simulink model "Offline_MiL_Sim_Public"  (R2024a)
settings: Solver=ode1  StartTime=0.0  StopTime=inf  FixedStep=step_size  RelTol=1e-3  EnableMultiTasking=on
PostLoadFcn:
  | if any(exist('dsrtsu_mdlpostloadfcn', 'file') ~= 0), dsrtsu_mdlpostloadfcn('Execute', bdroot); end
InitFcn:
  | , if any(exist('rtifpga_mdlclblib', 'file') ~= 0), rtifpga_mdlclblib('Init', bdroot); end,
  | , if any(exist('dsmpb_private', 'file') ~= 0), dsmpb_private('dsmpb_mdlclblib', 'Init', bdroot); end,
undefined symbols (not defined in the file or in its folder): Af, break_criteria, C_r, C_w, Cd, CurrentLosses, dens, DiscIntNeverNeededParam, FDR, fr, Friction, gain_Twr, grade_track, grav, IronLosses, Kp_c, lbh_ac, lbx_ac, lbx_ac_e, lbx_mhe, M_EM_acc_0, M_EM_acc_max, M_EM_brk_min, M_gen_max, M_mot_max, mpc_init_EM_acc, mpc_init_EM_brk, mpc_init_fric_brk, mps_kmh, Mv, n_0, n_em_max, n_gen_max, n_mot_max, n_vec, nout, numHiddenUnits, options, options_mhe, optparam, P, parameter_0, Q, R, r_dyn, R_w_c, R_w_e, R_w_r, rps_rpm, s_track, SE_selector_sim, start_distance_check, step_size, T_c, T_cool, T_e, T_init, T_max, t_mpc_on, T_r_0 ... (+21)
libraries: simulink x3, matrix_library x2, deeplib x1
(part 2 of 2)

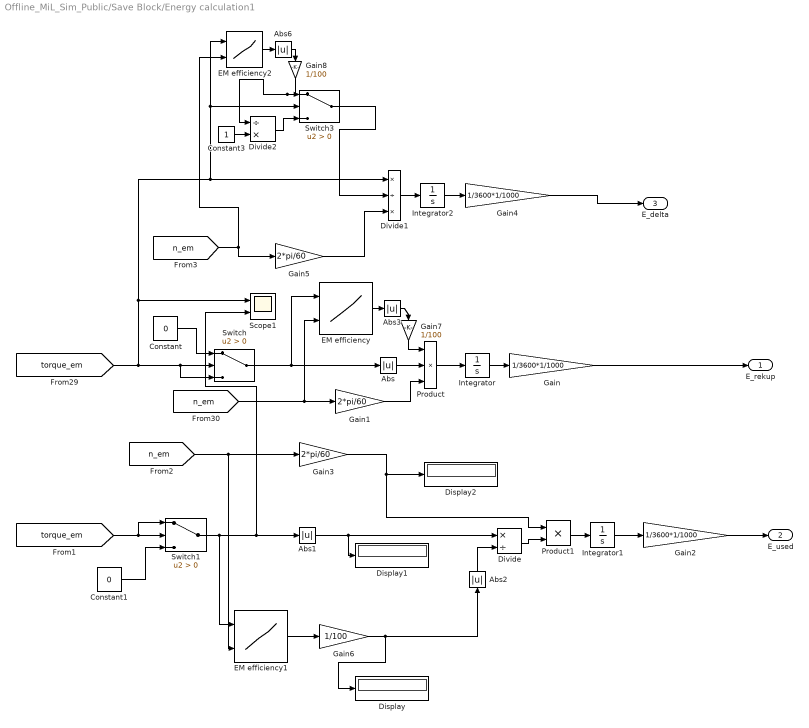
== system Offline_MiL_Sim_Public/Save Block/Energy calculation1 ==
  Abs{,1..3,6} (5 alike) : Abs  SaturateOnIntegerOverflow=off
  Constant : Constant  Value=0
  Constant1 : Constant  Value=0
  Constant3 : Constant
  Display : Display
  Display1 : Display
  Display2 : Display
  Divide : Product  Inputs=*/
  Divide1 : Product  Inputs=*/*
  Divide2 : Product  Inputs=/*
  EM efficiency : Lookup_n-D  BreakpointsForDimension1=data_efficiency(2:end,1)  BreakpointsForDimension2=data_efficiency(1,2:end)  Table=data_efficiency(2:end,2:end)  InternalRulePriority=Speed  RndMeth=Simplest
      settings: InputPortMap=u0,u1
  EM efficiency1 : Lookup_n-D  BreakpointsForDimension1=data_efficiency(2:end,1)  BreakpointsForDimension2=data_efficiency(1,2:end)  Table=data_efficiency(2:end,2:end)  InternalRulePriority=Speed  RndMeth=Simplest
      settings: InputPortMap=u0,u1
  EM efficiency2 : Lookup_n-D  BreakpointsForDimension1=data_efficiency(2:end,1)  BreakpointsForDimension2=data_efficiency(1,2:end)  Table=data_efficiency(2:end,2:end)  InternalRulePriority=Speed  RndMeth=Simplest
      settings: InputPortMap=u0,u1
  Gain : Gain  Gain=1/3600*1/1000
  Gain1 : Gain  Gain=2*pi/60
  Gain2 : Gain  Gain=1/3600*1/1000
  Gain3 : Gain  Gain=2*pi/60
  Gain4 : Gain  Gain=1/3600*1/1000
  Gain5 : Gain  Gain=2*pi/60
  Gain6 : Gain  Gain=1/100
  Gain7 : Gain  Gain=1/100
  Gain8 : Gain  Gain=1/100
  Integrator : Integrator
  Integrator1 : Integrator
  Integrator2 : Integrator
  Product : Product  Inputs=3
  Product1 : Product
  Scope1 : Scope  NumInputPorts=2
  Switch : Switch  Criteria=u2 > Threshold  SaturateOnIntegerOverflow=off  InputSameDT=off
  Switch1 : Switch  Criteria=u2 > Threshold  SaturateOnIntegerOverflow=off  InputSameDT=off
  Switch3 : Switch  Criteria=u2 > Threshold  SaturateOnIntegerOverflow=off  InputSameDT=off
  E_rekup : Outport  VectorParamsAs1DForOutWhenUnconnected=off
  E_used : Outport  Port=2  VectorParamsAs1DForOutWhenUnconnected=off
  E_delta : Outport  Port=3  VectorParamsAs1DForOutWhenUnconnected=off
  wires:
  Product/1 -> Integrator/1
  Switch/1 -> EM efficiency/1, Abs/1
  Gain1/1 -> Product/3
  Abs3/1 -> Gain7/1
  [n_em] -> Gain1/1, EM efficiency/2
  Abs/1 -> Product/2
  Constant/1 -> Switch/1
  Gain/1 -> E_rekup/1
  Integrator/1 -> Gain/1
  Divide/1 -> Product1/2
  Switch1/1 -> Scope1/2, Abs1/1, EM efficiency1/1
  [n_em] -> Gain3/1, EM efficiency1/2
  Abs1/1 -> Display1/1, Divide/1
  [torque_em] -> Switch1/1, Switch1/2
  Constant1/1 -> Switch1/3
  Gain2/1 -> E_used/1
  Integrator1/1 -> Gain2/1
  Product1/1 -> Integrator1/1
  Gain3/1 -> Product1/1, Display2/1
  Abs2/1 -> Divide/2
  EM efficiency/1 -> Abs3/1
  Integrator2/1 -> Gain4/1
  Gain4/1 -> E_delta/1
  Divide1/1 -> Integrator2/1
  [torque_em] -> Divide1/1, Switch3/2, EM efficiency2/1, Scope1/1, Switch/3, Switch/2
  [n_em] -> EM efficiency2/2, Gain5/1
  EM efficiency2/1 -> Abs6/1
  Gain5/1 -> Divide1/3
  Switch3/1 -> Divide1/2
  Abs6/1 -> Gain8/1
  Divide2/1 -> Switch3/3
  Constant3/1 -> Divide2/2
  Gain6/1 -> Display/1, Abs2/1
  EM efficiency1/1 -> Gain6/1
  Gain8/1 -> Divide2/1, Switch3/1
  Gain7/1 -> Product/1

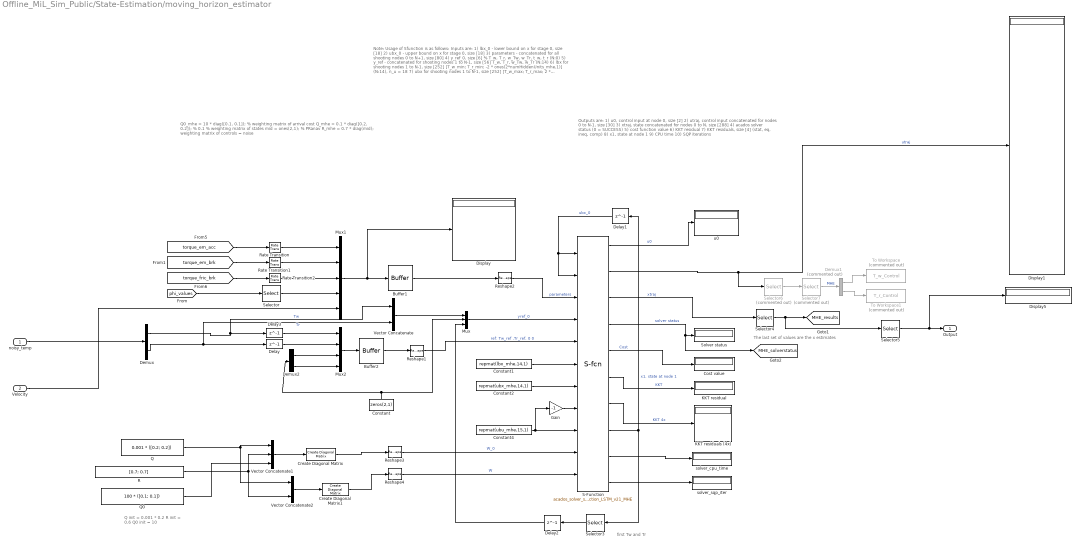
== system Offline_MiL_Sim_Public/State-Estimation/moving_horizon_estimator ==
  note: first Tw and Tr
  note: Q0_mhe = 10 * diag([0.1, 0.1]); % weighting matrix of arrival cost
      | Q_mhe = 0.1 * diag([0.2, 0.2]); % 0.1 % weighting matrix of states
      | mid = ones(2,1); % PRanav
      | R_mhe = 0.7 * diag(mid); weighting matrix of controls = noise
  note: Q init = 0.001 * 0.2
      | R init = 0.6
      | Q0 init = 10
  note: The last set of values are the x estimates
  note: Outputs are:
      | 1) u0, control input at node 0, size [2]
      | 2) utraj, control input concatenated for nodes 0 to N-1, size [30]
      | 3) xtraj, state concatenated for nodes 0 to N, size [288]
      | 4) acados solver status (0 = SUCCESS)
      | 5) cost function value
      | 6) KKT residual
      | 7) KKT residuals, size [4] (stat, eq, ineq, comp)
      | 8) x1, state at node 1
      | 9) CPU time
      | 10) SQP iterations
  note: Note: Usage of Sfunction is as follows:
      | Inputs are:
      | 1) lbx_0 - lower bound on x for stage 0, size [18]
      | 2) ubx_0 - upper bound on x for stage 0, size [18]
      | 3) parameters - concatenated for all shooting nodes 0 to N+1, size [80]
      | 4) y_ref_0, size [6]
      | % T_w, T_r, w_Tw, w_Tr, t_w, t_r (N:0)
      | 5) y_ref - concatenated for shooting nodes 1 to N-1, size [56]
      | T_w, T_r, w_Tw, w_Tr (N:14)
      | 6) lbx for shooting nodes 1 to N-1, size [252]
      | [T_w_min; T_r_min; -2 * ones(2*numHiddenUnits_mhe,1)] (N:14), n_u = 18
      | 7) ubx for shooting nodes 1 to N-1, size [252]
      | [T_w_max; T_r_max; 2 * ones(2*numHiddenUnits_mhe,1)] (N:14), n_u = 18
      | 8) lbu for shooting nodes 0 to N-1, size [30]
      | [0; 0] (N:15)
      | 9) ubu for shooting nodes 0 to N-1, size [30]
      | [100; 100] (N:15)
      | 10) cost_W_0 in column-major format, size [36]
      | blkdiag(Q_mhe, R_mhe, Q0_mhe)
      | 11) cost_W in column-major format, that is set for all intermediate shooting nodes: 1 to N-1, size [16]
      | blkdiag(Q_mhe, R_mhe)
  noisy_temp : Inport
  Velocity : Inport  Port=2
  Buffer1 : Buffer  N=(options_mhe.P+1)*options_mhe.n_parameter  V=((options_mhe.P+1)*options_mhe.n_parameter)-options_mhe.n_parameter  OutputFrames=off
  Buffer2 : Buffer  N=(options_mhe.P-1)*nout  V=(options_mhe.P-2)*nout  ic=repmat([60;60;0;0],13,1)  OutputFrames=off
  Constant : Constant  Value=zeros(2,1)
  Constant1 : Constant  Value=repmat(lbx_mhe,14,1)  SampleTime=options.Ts
  Constant2 : Constant  Value=repmat(ubx_mhe,14,1)  SampleTime=options.Ts
  Constant4 : Constant  Value=repmat(ubu_mhe,15,1)  SampleTime=options.Ts
  Cost value : Display
  Create Diagonal Matrix : matrix_library/Create Diagonal Matrix
      settings: LibrarySourceBlock=|
      | simulink/Matrix
      | Operations/Create Diagonal
      | Matrix
  Create Diagonal Matrix1 : matrix_library/Create Diagonal Matrix
      settings: LibrarySourceBlock=|
      | simulink/Matrix
      | Operations/Create Diagonal
      | Matrix
  Delay : Delay  DelayLength=1  InitialCondition=60
  Delay1 : Delay  DelayLength=1  InitialCondition=options_mhe.x0
  Delay2 : Delay  DelayLength=1  InitialCondition=[60;60]
  Delay3 : Delay  DelayLength=1  InitialCondition=60
  Demux : Demux  Outputs=2
  Demux1 : Demux  Commented=on  Outputs=2
  Demux2 : Demux  Outputs=2
  Display : Display
  Display1 : Display
  Display5 : Display
  Gain : Gain  Gain=-1
  KKT residual : Display
  KKT residuals (4x) : Display
  Mux : Mux  Inputs=3
  Mux1 : Mux  Inputs=5
  Mux2 : Mux
  Q : Constant  Value=0.001 * ([0.2; 0.2])  VectorParams1D=off
  Q0 : Constant  Value=100 * ([0.1; 0.1])
  R : Constant  Value=[0.7; 0.7]
  Rate Transition : RateTransition  OutPortSampleTime=options_mhe.Ts
  Rate Transition1 : RateTransition  OutPortSampleTime=options_mhe.Ts
  Rate Transition2 : RateTransition  OutPortSampleTime=options_mhe.Ts
  Reshape{1..4} (4 alike) : Reshape
  S-Function : S-Function  FunctionName=acados_solver_sfunction_LSTM_v21_MHE  SFunctionDeploymentMode=off  EnableBusSupport=off
  Selector : Selector  InputPortWidth=41  IndexOptions=Index vector (dialog)  Indices=1  OutputSizes=1
  Selector3 : Selector  InputPortWidth=2+(numHiddenUnits*2)  IndexOptions=Index vector (dialog)  Indices=[1 2]  OutputSizes=1
  Selector4 : Selector  InputPortWidth=288  IndexOptions=Index vector (dialog)  Indices=[(18*15)+1:18*16]  OutputSizes=1
  Selector5 : Selector  InputPortWidth=18  IndexOptions=Index vector (dialog)  Indices=[1 2]  OutputSizes=1
  Selector6 : Selector  Commented=on  InputPortWidth=18*15  IndexOptions=Index vector (dialog)  Indices=[(18*14)+1:18*15]  OutputSizes=1
  Selector7 : Selector  Commented=on  InputPortWidth=18  IndexOptions=Index vector (dialog)  Indices=[1:2]  OutputSizes=1
  Solver status : Display
  To Workspace : ToWorkspace  Commented=on  VariableName=T_w_Control  SampleTime=-1
      settings: Save2DSignal=2-D array (concatenate along first dimension)
  To Workspace1 : ToWorkspace  Commented=on  VariableName=T_r_Control  SampleTime=-1
      settings: Save2DSignal=2-D array (concatenate along first dimension)
  Vector Concatenate : Concatenate
  Vector Concatenate1 : Concatenate  NumInputs=3
  Vector Concatenate2 : Concatenate
  solver_cpu_time : Display
  solver_sqp_iter : Display
  u0 : Display
  Output : Outport
  tag scope: MHE_results=global, MHE_solverstatus=global
  wires:
  [torque_fric_brk] -> Rate Transition2/1
  Mux/1 -> S-Function/4  "yref_0"
  [torque_em_brk] -> Rate Transition1/1
  S-Function/2 -> Display1/1, Selector6/1  "utraj"
  R/1 -> Vector Concatenate1/2, Vector Concatenate2/2
  Velocity/1 -> Mux1/5
  Q0/1 -> Vector Concatenate1/3
  Create Diagonal Matrix1/1 -> Reshape4/1
  S-Function/3 -> Selector4/1  "xtraj"
  noisy_temp/1 -> Demux/1
  [phi_values] -> Selector/1
  Rate Transition2/1 -> Mux1/3
  Demux/2 -> Vector Concatenate/2, Delay/1  "Tr"
  Create Diagonal Matrix/1 -> Reshape3/1
  Buffer1/1 -> Reshape2/1
  Q/1 -> Vector Concatenate1/1, Vector Concatenate2/1
  Vector Concatenate1/1 -> Create Diagonal Matrix/1
  Delay1/1 -> S-Function/2, S-Function/1  "ubx_0"
  Vector Concatenate/1 -> Mux/1
  S-Function/1 -> u0/1  "u0"
  Selector4/1 -> Selector5/1, [MHE_results]
  Demux/1 -> Delay3/1, Vector Concatenate/1  "Tw"
  Vector Concatenate2/1 -> Create Diagonal Matrix1/1
  Reshape2/1 -> S-Function/3  "parameters"
  [torque_em_acc] -> Rate Transition/1
  Rate Transition/1 -> Mux1/1
  Rate Transition1/1 -> Mux1/2
  S-Function/4 -> [MHE_solverstatus], Solver status/1  "solver status"
  Mux1/1 -> Display/1, Buffer1/1
  Selector/1 -> Mux1/4
  Selector5/1 -> Display5/1, Output/1
  Selector6/1 -> Selector7/1
  Selector7/1 -> Demux1/1  "MHE"
  Demux1/1 -> To Workspace/1
  Demux1/2 -> To Workspace1/1
  Reshape4/1 -> S-Function/11  "W"
  Reshape3/1 -> S-Function/10  "W_0"
  Constant1/1 -> S-Function/6
  Constant2/1 -> S-Function/7
  Constant4/1 -> S-Function/9, Gain/1
  Reshape1/1 -> S-Function/5  "ref: Tw_ref ,Tr_ref, 0 0"
  Demux2/1 -> Mux2/3
  Demux2/2 -> Mux2/4
  Delay/1 -> Mux2/2
  Delay3/1 -> Mux2/1
  Mux2/1 -> Buffer2/1
  Buffer2/1 -> Reshape1/1
  S-Function/10 -> solver_sqp_iter/1
  S-Function/9 -> solver_cpu_time/1
  S-Function/5 -> Cost value/1  "Cost"
  S-Function/8 -> Delay1/1, Selector3/1  "x1, state at node 1"
  S-Function/6 -> KKT residual/1  "KKT"
  S-Function/7 -> KKT residuals (4x)/1  "KKT 4x"
  Delay2/1 -> Mux/3
  Constant/1 -> Demux2/1, Mux/2
  Selector3/1 -> Delay2/1
  Gain/1 -> S-Function/8

== system Offline_MiL_Sim_Public/Vehicle Model/Driver Model ==
  note: source: Jinming Liu, Modeling, Configuration and control optimization of power split hybrid vehiclesm, Dissertation, 2007
  v_veh (km/h) : Inport
  v_des (km/h) : Inport  Port=2
  "-1 to 1 " : Saturate  UpperLimit=1  LowerLimit=-1
  1/Ti_c : Gain  Gain=1/Ti_c  SaturateOnIntegerOverflow=on  OutDataTypeStr=Inherit: Same as input  ParamDataTypeStr=Inherit: Same as input
  1/Tt_c : Gain  Gain=1/Tt_c  SaturateOnIntegerOverflow=on  OutDataTypeStr=Inherit: Same as input  ParamDataTypeStr=Inherit: Same as input
  Integrator1 : Integrator
  Kp_c : Gain  Gain=Kp_c  SaturateOnIntegerOverflow=on  OutDataTypeStr=Inherit: Same as input  ParamDataTypeStr=Inherit: Same as input
  Normalize : Gain  Gain=1/v_max_c  SaturateOnIntegerOverflow=on  OutDataTypeStr=Inherit: Same as input  ParamDataTypeStr=Inherit: Same as input
  Normalize1 : Gain  Gain=1/v_max_c  SaturateOnIntegerOverflow=on  OutDataTypeStr=Inherit: Same as input  ParamDataTypeStr=Inherit: Same as input
  Sum1 : Sum  InputSameDT=on  SaturateOnIntegerOverflow=on  OutDataTypeStr=Inherit: Same as first input
  Sum5 : Sum  Inputs=-+  InputSameDT=on  SaturateOnIntegerOverflow=on  OutDataTypeStr=Inherit: Same as first input
  Sum7 : Sum  Inputs=+-  InputSameDT=on  SaturateOnIntegerOverflow=on  OutDataTypeStr=Inherit: Same as first input
  Sum8 : Sum  InputSameDT=on  SaturateOnIntegerOverflow=on  OutDataTypeStr=Inherit: Same as first input
  driver_cmd : Outport  VectorParamsAs1DForOutWhenUnconnected=off
  wires:
  Normalize/1 -> Sum7/1
  v_veh (km/h)/1 -> Normalize1/1  "v_ist"
  v_des (km/h)/1 -> Normalize/1  "vdes"
  Sum5/1 -> 1/Tt_c/1
  "-1 to 1 "/1 -> Sum5/2, driver_cmd/1
  Integrator1/1 -> Sum1/2
  1/Ti_c/1 -> Sum8/1
  Sum8/1 -> Integrator1/1
  1/Tt_c/1 -> Sum8/2
  Kp_c/1 -> 1/Ti_c/1, Sum1/1
  Sum1/1 -> "-1 to 1 "/1, Sum5/1
  Sum7/1 -> Kp_c/1
  Normalize1/1 -> Sum7/2

== system Offline_MiL_Sim_Public/Vehicle Model/LSTM-Based Thermal Model grad ==
  Rotational_Speed [rpm] : Inport
  Torque_EM [Nm] : Inport  Port=2
  Constant3 : Constant  Value=YMin_mhe
  Constant4 : Constant  Value=T_cool
  Delay : Delay  DelayLength=1  InitialCondition=[T_w_0;T_r_0]
  Demux4 : Demux  Outputs=2
  Demux5 : Demux  Commented=on  Outputs=2
  Discrete-Time Integrator : DiscreteIntegrator  gainval=1  InitialCondition=[T_w_0;T_r_0]  SampleTime=-1  ICPrevOutput=DiscIntNeverNeededParam  ICPrevScaledInput=DiscIntNeverNeededParam
  From1 : From  Commented=on  GotoTag=T_wr  TagVisibility=global
  Gain2 : Gain  Gain=1/n_em_max
  Gain3 : Gain  Gain=1/M_EM_acc_max
  Gain6 : Gain  Gain=YMax_mhe-YMin_mhe
  Gain7 : Gain  Gain=1/(T_max-T_cool)
  Gain8 : Gain  Gain=1/(T_max-T_cool)
  Mux : Mux
  Reshape : Reshape  OutputDimensionality=Customize  OutputDimensions=[4,1]
  Stateful Predict : deeplib/Stateful Predict  Network=Network from MAT-file  NetworkFunction=untitled  NetworkFilePath=e_Sim\LSTM_8HU_10000ep_grad_slx.mat  InputDataFormats={ '', '' }  SampleTime=-1  ForceInterpretedSim=off  EnableDLNetwork=on  LastKnownNetworkFilePath=''  LastKnownNetworkTimeStamp=''
  Sum2 : Sum  Inputs=|++
  Sum3 : Sum  Inputs=-+|
  Sum4 : Sum  Inputs=-+|
  To Workspace17 : ToWorkspace  VariableName=XTest  SaveFormat=Timeseries  SampleTime=-1
  To Workspace18 : ToWorkspace  VariableName=YPred  SaveFormat=Timeseries  SampleTime=-1
  T_w_LSTM [°C] : Outport
  T_r_LSTM [°C] : Outport  Port=2
  wires:
  Mux/1 -> Reshape/1
  Demux5/1 -> ?
  Rotational_Speed [rpm]/1 -> Gain2/1
  Torque_EM [Nm]/1 -> Gain3/1
  Gain7/1 -> Mux/3
  Sum4/1 -> Gain8/1
  Stateful Predict/1 -> Gain6/1
  Constant4/1 -> Sum4/1, Sum3/1
  Gain8/1 -> Mux/4
  Sum3/1 -> Gain7/1
  Gain2/1 -> Mux/1
  Demux5/2 -> ?
  Demux4/2 -> Sum4/2, T_r_LSTM [°C]/1
  Delay/1 -> Demux4/1
  Constant3/1 -> Sum2/2
  Demux4/1 -> Sum3/2, T_w_LSTM [°C]/1
  Sum2/1 -> Discrete-Time Integrator/1, To Workspace18/1
  From1/1 -> Demux5/1
  Discrete-Time Integrator/1 -> Delay/1
  Gain3/1 -> Mux/2
  Gain6/1 -> Sum2/1
  Reshape/1 -> Stateful Predict/1, To Workspace17/1

== system Offline_MiL_Sim_Public/Vehicle Model/Thermal Model DENSO ==
  "SpeedIn " : Inport
  TorqueIn : Inport  Port=2
  Ground : Ground
  Terminator : Terminator
  Terminator1 : Terminator
  T_wr : Outport
  T_wr_muxed : Outport  Port=2
  wires:
  TorqueIn/1 -> Terminator/1  "TorqueIn"
  "SpeedIn "/1 -> Terminator1/1
  Ground/1 -> T_wr_muxed/1, T_wr/1

== system Offline_MiL_Sim_Public/Vehicle Model/Thermisches Modell EM - LPTN ==
  Drehzahl_rpm : Inport
  Torque_Nm : Inport  Port=2
  Abs : Abs  SaturateOnIntegerOverflow=off
  Coolant Temp : Constant  Value=T_c  VectorParams1D=off
  Demux : Demux  Outputs=2
  Demux1 : Demux  Outputs=2
  Demux2 : Demux  Outputs=2
  Display : Display
  Display1 : Display
  Display2 : Display
  Environment Temp : Constant  Value=T_e  VectorParams1D=off
  Gain1 : Gain  Gain=0.8
  Gain2 : Gain  Gain=0.2
  Goto : Goto  Commented=on  GotoTag=R_w_r  TagVisibility=global
  Goto1 : Goto  Commented=on  GotoTag=R_r_e  TagVisibility=global
  K->C : Constant  Value=273.15
  "LPTN Model " : Subsystem
  Mux : Mux  Inputs=2
  Mux1 : Mux
  Parameter Calculation : Subsystem  Commented=on
  Subsystem1 : Subsystem
  Subsystem2 : Subsystem
  Subsystem3 : Subsystem
  Sum : Sum  Inputs=|++
  Sum1 : Sum  Inputs=++|
  Sum5 : Sum  Inputs=|+-
  Temperaturen_C : Outport  VectorParamsAs1DForOutWhenUnconnected=off
  wires:
  Demux/1 -> Subsystem3/1(torque)  "torque"
  Demux/2 -> Subsystem3/2(speed)  "speed"
  Demux2/1 -> Subsystem2/1(torque)  "torque"
  Demux2/2 -> Subsystem2/2(speed)  "speed"
  Demux1/1 -> Subsystem1/1(torque)  "torque"
  Demux1/2 -> Subsystem1/2(speed)  "speed"
  Subsystem3/1(iron loss) -> Sum/1
  Sum1/1 -> Display1/1, Mux1/2  "P_R"
  Subsystem2/1(friction loss) -> Sum1/2
  Gain2/1 -> Sum1/1
  Gain1/1 -> Sum/2
  Sum/1 -> Display/1, Mux1/1  "P_W"
  Coolant Temp/1 -> Mux1/3
  Environment Temp/1 -> Mux1/4
  Mux1/1 -> "LPTN Model "/1(1:Pw 2: Pr 3:Tc  4:Te)
  "LPTN Model "/1("1:Tw, 2:Tr") -> Sum5/1  "[K]"
  Subsystem1/1(iron loss) -> Gain1/1, Gain2/1
  Drehzahl_rpm/1 -> Mux/2
  Mux/1 -> Demux2/1, Demux1/1, Demux/1
  K->C/1 -> Sum5/2
  Sum5/1 -> Display2/1, Temperaturen_C/1  "[gradC]"
  Parameter Calculation/1(R_w_r) -> Goto/1
  Parameter Calculation/2(R_r_e) -> Goto1/1
  Torque_Nm/1 -> Abs/1
  Abs/1 -> Mux/1

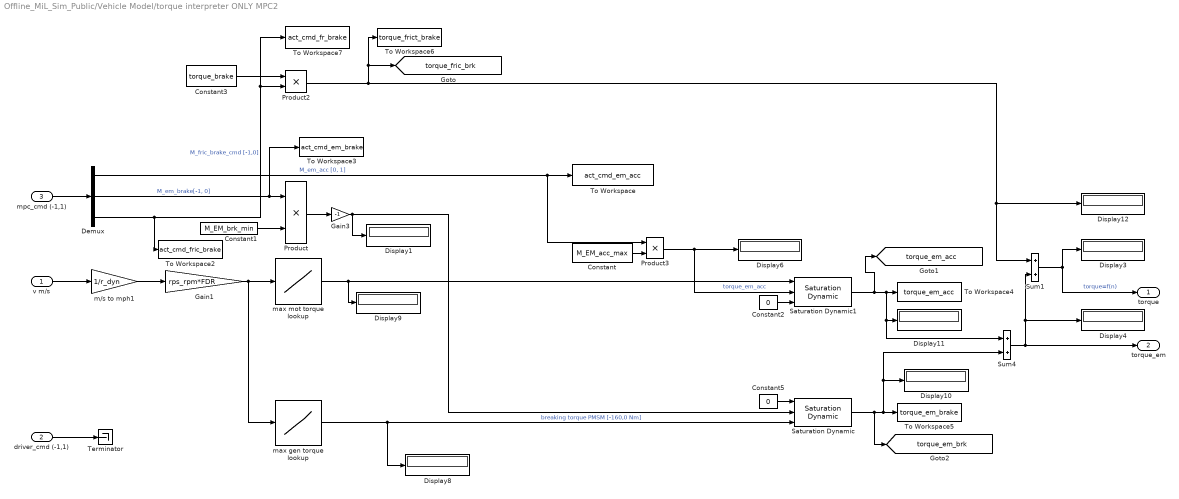
== system Offline_MiL_Sim_Public/Vehicle Model/torque interpreter ONLY MPC2 ==
  v m/s : Inport
  driver_cmd (-1,1) : Inport  Port=2
  mpc_cmd (-1,1) : Inport  Port=3
  Constant : Constant  Value=M_EM_acc_max
  Constant1 : Constant  Value=M_EM_brk_min
  Constant2 : Constant  Value=0
  Constant3 : Constant  Value=torque_brake
  Constant5 : Constant  Value=0
  Demux : Demux  Outputs=3
  Display{1,3..4,6,8..12} (9 alike) : Display
  Gain1 : Gain  Gain=rps_rpm*FDR
  Gain3 : Gain  Gain=-1
  Product : Product
  Product2 : Product
  Product3 : Product
  Saturation Dynamic : simulink/Discontinuities/Saturation Dynamic  OutMin=[]  OutMax=[]  OutDataTypeStr=Inherit: Same as second input  OutDataType=fixdt(1, 16)  OutScaling=2^-10  DoSatur=off
  Saturation Dynamic1 : simulink/Discontinuities/Saturation Dynamic  OutMin=[]  OutMax=[]  OutDataTypeStr=Inherit: Same as second input  OutDataType=fixdt(1, 16)  OutScaling=2^-10  DoSatur=off
  Sum1 : Sum
  Sum4 : Sum
  Terminator : Terminator
  To Workspace : ToWorkspace  VariableName=act_cmd_em_acc  SampleTime=-1
      settings: Save2DSignal=2-D array (concatenate along first dimension)
  To Workspace2 : ToWorkspace  VariableName=act_cmd_fric_brake  SampleTime=-1
      settings: Save2DSignal=2-D array (concatenate along first dimension)
  To Workspace3 : ToWorkspace  VariableName=act_cmd_em_brake  SampleTime=-1
      settings: Save2DSignal=2-D array (concatenate along first dimension)
  To Workspace4 : ToWorkspace  VariableName=torque_em_acc  SampleTime=-1
      settings: Save2DSignal=2-D array (concatenate along first dimension)
  To Workspace5 : ToWorkspace  VariableName=torque_em_brake  SampleTime=-1
      settings: Save2DSignal=2-D array (concatenate along first dimension)
  To Workspace6 : ToWorkspace  VariableName=torque_frict_brake  SampleTime=-1
      settings: Save2DSignal=2-D array (concatenate along first dimension)
  To Workspace7 : ToWorkspace  VariableName=act_cmd_fr_brake  SampleTime=-1
      settings: Save2DSignal=2-D array (concatenate along first dimension)
  m/s to mph1 : Gain  Gain=1/r_dyn  SaturateOnIntegerOverflow=on  OutDataTypeStr=Inherit: Same as input  ParamDataTypeStr=Inherit: Same as input
  max gen torque lookup : Lookup_n-D  NumberOfTableDimensions=1  BreakpointsForDimension1=n_gen_max  Table=M_gen_max  InternalRulePriority=Speed  RndMeth=Simplest
  max mot torque lookup : Lookup_n-D  NumberOfTableDimensions=1  BreakpointsForDimension1=n_mot_max  Table=M_mot_max  InternalRulePriority=Speed  RndMeth=Simplest
  torque : Outport  VectorParamsAs1DForOutWhenUnconnected=off
  torque_em : Outport  Port=2  VectorParamsAs1DForOutWhenUnconnected=off
  tag scope: torque_em_acc=global, torque_em_brk=global, torque_fric_brk=global
  wires:
  v m/s/1 -> m/s to mph1/1
  m/s to mph1/1 -> Gain1/1
  Sum1/1 -> torque/1, Display3/1  "torque=f(n)"
  Gain1/1 -> max mot torque lookup/1, max gen torque lookup/1
  max gen torque lookup/1 -> Display8/1, Saturation Dynamic/3  "breaking torque PMSM [-160,0 Nm]"
  Demux/1 -> Product3/1, To Workspace/1  "M_em_acc [0, 1]"
  Demux/2 -> To Workspace3/1, Product/1  "M_em_brake[-1, 0]"
  Demux/3 -> To Workspace7/1, Product2/2, To Workspace2/1  "M_fric_brake_cmd [-1,0]"
  mpc_cmd (-1,1)/1 -> Demux/1
  Constant3/1 -> Product2/1
  Saturation Dynamic/1 -> To Workspace5/1, Display10/1, Sum4/2, [torque_em_brk]
  Constant5/1 -> Saturation Dynamic/1
  Sum4/1 -> Sum1/2, Display4/1, torque_em/1
  Product/1 -> Gain3/1
  driver_cmd (-1,1)/1 -> Terminator/1
  Constant/1 -> Product3/2
  Constant1/1 -> Product/2
  Saturation Dynamic1/1 -> Sum4/1, Display11/1, To Workspace4/1, [torque_em_acc]
  Constant2/1 -> Saturation Dynamic1/3
  Product3/1 -> Saturation Dynamic1/2, Display6/1  "torque_em_acc"
  max mot torque lookup/1 -> Display9/1, Saturation Dynamic1/1
  Gain3/1 -> Display1/1, Saturation Dynamic/2
  Product2/1 -> [torque_fric_brk], To Workspace6/1, Sum1/1, Display12/1

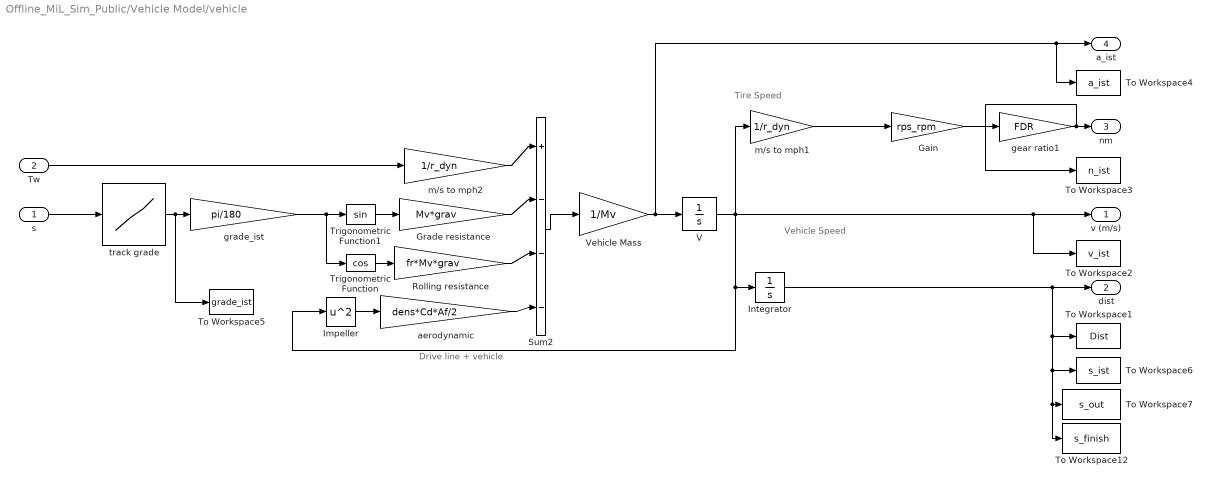
== system Offline_MiL_Sim_Public/Vehicle Model/vehicle ==
  note: Drive line + vehicle
  note: Vehicle Speed
  note: Tire Speed
  s : Inport
  Tw : Inport  Port=2
  Gain : Gain  Gain=rps_rpm
  Grade resistance : Gain  Gain=Mv*grav  SaturateOnIntegerOverflow=on  OutDataTypeStr=Inherit: Same as input  ParamDataTypeStr=Inherit: Same as input
  Impeller : Math  Operator=square  SignedPower=on
  Integrator : Integrator
  Rolling resistance : Gain  Gain=fr*Mv*grav  SaturateOnIntegerOverflow=on  OutDataTypeStr=Inherit: Same as input  ParamDataTypeStr=Inherit: Same as input
  Sum2 : Sum  Inputs=|+|-|-|-  InputSameDT=on  SaturateOnIntegerOverflow=on  OutDataTypeStr=Inherit: Same as first input
  To Workspace1 : ToWorkspace  VariableName=Dist  SampleTime=-1
  To Workspace12 : ToWorkspace  VariableName=s_finish  SampleTime=-1
      settings: MaxDataPoints=1  Save2DSignal=2-D array (concatenate along first dimension)
  To Workspace2 : ToWorkspace  VariableName=v_ist  SampleTime=-1
  To Workspace3 : ToWorkspace  VariableName=n_ist  SampleTime=-1
  To Workspace4 : ToWorkspace  VariableName=a_ist  SampleTime=-1
  To Workspace5 : ToWorkspace  VariableName=grade_ist  SampleTime=-1
  To Workspace6 : ToWorkspace  VariableName=s_ist  SampleTime=-1
  To Workspace7 : ToWorkspace  VariableName=s_out  SampleTime=-1
      settings: Save2DSignal=2-D array (concatenate along first dimension)
  Trigonometric Function : Trigonometry  Operator=cos
  Trigonometric Function1 : Trigonometry
  V : Integrator  InitialCondition=v_0  LimitOutput=on  UpperSaturationLimit=v_max * mps_kmh  LowerSaturationLimit=0
  Vehicle Mass : Gain  Gain=1/Mv  SaturateOnIntegerOverflow=on  OutDataTypeStr=Inherit: Same as input  ParamDataTypeStr=Inherit: Same as input
  aerodynamic : Gain  Gain=dens*Cd*Af/2  SaturateOnIntegerOverflow=on  OutDataTypeStr=Inherit: Same as input  ParamDataTypeStr=Inherit: Same as input
  gear ratio1 : Gain  Gain=FDR
  grade_ist : Gain  Gain=pi/180  SaturateOnIntegerOverflow=on  OutDataTypeStr=Inherit: Same as input  ParamDataTypeStr=Inherit: Same as input
  m/s to mph1 : Gain  Gain=1/r_dyn  SaturateOnIntegerOverflow=on  OutDataTypeStr=Inherit: Same as input  ParamDataTypeStr=Inherit: Same as input
  m/s to mph2 : Gain  Gain=1/r_dyn  SaturateOnIntegerOverflow=on  OutDataTypeStr=Inherit: Same as input  ParamDataTypeStr=Inherit: Same as input
  track grade : Lookup_n-D  NumberOfTableDimensions=1  BreakpointsForDimension1=s_track  Table=grade_track  InternalRulePriority=Speed  RndMeth=Simplest
  v (m/s) : Outport  InitialOutput=0  VectorParamsAs1DForOutWhenUnconnected=off
  dist : Outport  Port=2  InitialOutput=0  VectorParamsAs1DForOutWhenUnconnected=off
  nm : Outport  Port=3  InitialOutput=0  VectorParamsAs1DForOutWhenUnconnected=off
  a_ist : Outport  Port=4  InitialOutput=0  VectorParamsAs1DForOutWhenUnconnected=off
  wires:
  Trigonometric Function/1 -> Rolling resistance/1
  Trigonometric Function1/1 -> Grade resistance/1
  Impeller/1 -> aerodynamic/1
  m/s to mph1/1 -> Gain/1
  aerodynamic/1 -> Sum2/4
  Rolling resistance/1 -> Sum2/3
  Grade resistance/1 -> Sum2/2
  V/1 -> Impeller/1, Integrator/1, To Workspace2/1, v (m/s)/1, m/s to mph1/1
  grade_ist/1 -> Trigonometric Function/1, Trigonometric Function1/1
  Sum2/1 -> Vehicle Mass/1
  Vehicle Mass/1 -> To Workspace4/1, a_ist/1, V/1
  Tw/1 -> m/s to mph2/1
  m/s to mph2/1 -> Sum2/1
  gear ratio1/1 -> To Workspace3/1, nm/1
  Gain/1 -> gear ratio1/1
  track grade/1 -> To Workspace5/1, grade_ist/1
  s/1 -> track grade/1
  Integrator/1 -> To Workspace12/1, To Workspace7/1, To Workspace6/1, To Workspace1/1, dist/1

== system Offline_MiL_Sim_Public/MPC/Pred_Traj_and_costs_calc/Subsystem ==
  v : Inport
  v_ref : Inport  Port=2
  u : Inport  Port=3
  dt_u : Inport  Port=4
  Constant : Constant  Value=Q(3,3)
  Constant1 : Constant  Value=R(1,1)
  Constant2 : Constant  Value=U(1,1)
  Constant3 : Constant  Value=options.P
  MATLAB Function : MATLAB Function  TreatAsAtomicUnit=on
  To Workspace : ToWorkspace  VariableName=cost_v  SampleTime=-1
  To Workspace1 : ToWorkspace  VariableName=cost_u  SampleTime=-1
  To Workspace2 : ToWorkspace  VariableName=cost_du  SampleTime=-1
  To Workspace3 : ToWorkspace  VariableName=cost_traj  SampleTime=-1
  cost : Outport  VectorParamsAs1DForOutWhenUnconnected=off
  wires:
  MATLAB Function/1(cost) -> cost/1
  dt_u/1 -> MATLAB Function/4(dt_u)
  v/1 -> MATLAB Function/1(v)
  u/1 -> MATLAB Function/3(u)
  v_ref/1 -> MATLAB Function/2(v_ref)
  Constant/1 -> MATLAB Function/5(Q)
  Constant2/1 -> MATLAB Function/7(U)
  Constant1/1 -> MATLAB Function/6(R)
  MATLAB Function/4(cost_U) -> To Workspace2/1
  MATLAB Function/3(cost_R) -> To Workspace1/1
  MATLAB Function/2(cost_Q) -> To Workspace/1
  MATLAB Function/5(cost_traj) -> To Workspace3/1
  Constant3/1 -> MATLAB Function/8(P)

== system Offline_MiL_Sim_Public/Vehicle Model/Thermisches Modell EM - LPTN/LPTN Model  ==
  1:Pw 2: Pr 3:Tc  4:Te : Inport
  Constant : Constant  Value=R_w_r
  Constant1 : Constant  Value=R_w_r
  Constant2 : Constant  Value=R_w_e
  Demux : Demux
  Divide : Product  Inputs=*/
  Divide1 : Product  Inputs=*/
  Divide2 : Product  Inputs=*/
  Integrator : Integrator  InitialCondition=T_init(1)
  Integrator2 : Integrator  InitialCondition=T_init(2)
  Mux : Mux  Inputs=2
  Sum{,1,3..4,7,9} (6 alike) : Sum  Inputs=|+-
  Sum2 : Sum  Inputs=+++
  Sum5 : Sum  Inputs=+-|
  Sum6 : Sum
  gain : Gain  Gain=1/C_w
  gain1 : Gain  Gain=1/C_r
  gain3 : Gain  Gain=1/R_w_e
  gain4 : Gain  Gain=1/R_w_c
  "1:Tw, 2:Tr" : Outport  VectorParamsAs1DForOutWhenUnconnected=off
  wires:
  1:Pw 2: Pr 3:Tc  4:Te/1 -> Demux/1
  Demux/1 -> Sum/1  "Pw"
  Demux/2 -> Sum9/1  "Pr"
  Sum3/1 -> gain3/1  "Tw-Te"
  Sum4/1 -> Divide/1  "Tw-Tr"
  Integrator2/1 -> Sum5/1, Sum7/1, Mux/2, Sum4/2  "Tr"
  Divide/1 -> Sum2/1
  gain3/1 -> Sum2/2
  Sum1/1 -> gain4/1  "Tw-Tc"
  gain4/1 -> Sum2/3
  Sum/1 -> gain/1
  gain/1 -> Integrator/1  "dt/t Tw"
  Demux/4 -> Sum7/2, Sum3/2  "T_e"
  Demux/3 -> Sum1/2  "T_c"
  Sum7/1 -> Divide2/1  "Tr-Te"
  Sum5/1 -> Divide1/1  "Tr-Tw"
  Divide1/1 -> Sum6/1
  Divide2/1 -> Sum6/2
  Sum9/1 -> gain1/1
  gain1/1 -> Integrator2/1  "dt/t Tr"
  Sum6/1 -> Sum9/2
  Mux/1 -> "1:Tw, 2:Tr"/1
  Constant1/1 -> Divide1/2
  Constant2/1 -> Divide2/2
  Constant/1 -> Divide/2
  Sum2/1 -> Sum/2
  Integrator/1 -> Sum1/1, Sum3/1, Sum4/1, Mux/1, Sum5/2  "Tw"

== system Offline_MiL_Sim_Public/Vehicle Model/Thermisches Modell EM - LPTN/Parameter Calculation ==
  n /rpm : Inport
  1-D Lookup Table : Lookup_n-D  NumberOfTableDimensions=1  BreakpointsForDimension1=n_vec  Table=optparam(:,2)  InternalRulePriority=Speed  RndMeth=Simplest
  1-D Lookup Table1 : Lookup_n-D  NumberOfTableDimensions=1  BreakpointsForDimension1=n_vec  Table=optparam(:,4)  InternalRulePriority=Speed  RndMeth=Simplest
  R_w_r : Outport  VectorParamsAs1DForOutWhenUnconnected=off
  R_r_e : Outport  Port=2  VectorParamsAs1DForOutWhenUnconnected=off
  wires:
  n /rpm/1 -> 1-D Lookup Table1/1, 1-D Lookup Table/1
  1-D Lookup Table/1 -> R_w_r/1
  1-D Lookup Table1/1 -> R_r_e/1

== system Offline_MiL_Sim_Public/Vehicle Model/Thermisches Modell EM - LPTN/Subsystem1 ==
  torque : Inport
  speed : Inport  Port=2
  Abs : Abs  SaturateOnIntegerOverflow=off
  IronLosses : Lookup_n-D  Commented=on  BreakpointsForDimension1=IronLosses.Torque  BreakpointsForDimension2=IronLosses.RotSpeed  Table=IronLosses.Losses  InternalRulePriority=Speed  RndMeth=Simplest
      settings: InputPortMap=u0,u1
  MATLAB Function : MATLAB Function  TreatAsAtomicUnit=on
  iron loss : Outport  VectorParamsAs1DForOutWhenUnconnected=off
  wires:
  MATLAB Function/1(P_Iron_Mot) -> iron loss/1
  speed/1 -> MATLAB Function/1(speed)
  torque/1 -> Abs/1
  Abs/1 -> MATLAB Function/2(torque)

== system Offline_MiL_Sim_Public/Vehicle Model/Thermisches Modell EM - LPTN/Subsystem2 ==
  torque : Inport
  speed : Inport  Port=2
  FrictionLosses : Lookup_n-D  Commented=on  BreakpointsForDimension1=Friction.Torque  BreakpointsForDimension2=Friction.RotSpeed  Table=Friction.Losses  InternalRulePriority=Speed  RndMeth=Simplest
      settings: InputPortMap=u0,u1
  MATLAB Function : MATLAB Function  TreatAsAtomicUnit=on
  friction loss : Outport  VectorParamsAs1DForOutWhenUnconnected=off
  wires:
  speed/1 -> MATLAB Function/1(speed)
  MATLAB Function/1(P_Frict_Mot) -> friction loss/1
  torque/1 -> MATLAB Function/2(torque)

== system Offline_MiL_Sim_Public/Vehicle Model/Thermisches Modell EM - LPTN/Subsystem3 ==
  torque : Inport
  speed : Inport  Port=2
  Abs : Abs  SaturateOnIntegerOverflow=off
  CurrentLosses : Lookup_n-D  Commented=on  BreakpointsForDimension1=CurrentLosses.Torque  BreakpointsForDimension2=CurrentLosses.RotSpeed  Table=CurrentLosses.Losses  InternalRulePriority=Speed  RndMeth=Simplest
      settings: InputPortMap=u0,u1
  MATLAB Function : MATLAB Function  TreatAsAtomicUnit=on
  iron loss : Outport  VectorParamsAs1DForOutWhenUnconnected=off
  wires:
  torque/1 -> Abs/1
  speed/1 -> MATLAB Function/1(speed)
  MATLAB Function/1(P_Current_Mot) -> iron loss/1
  Abs/1 -> MATLAB Function/2(torque)

== matlab function Offline_MiL_Sim_Public/MPC/MATLAB Function1 ==
  data: phi input; par_traj_merged output; v_r input; P input
function par_traj_merged = get_par_traj(phi,v_r,P)
%#codegen
%     y_ref_merged = zeros(150,1);
%     y_ref_merged = zeros(P*(n_controls-2+n_states),1);
    j = 1;
    % Depended on: y _ [v, M_EM_acc, M_EM_brk, M-fric_brk];
    
    par_traj_merged = zeros(160,1);
    for i=1:(P+1) % (or until P+1)
        par_traj_merged(j) = phi(i); % v
        j = j+1;
        if i == (P+1)
            par_traj_merged(j) = v_r(i-1); % u1
        else
            par_traj_merged(j) = v_r(i); % u1
        end
        j = j+1;
%         y_ref_merged(j) = x(i); % v
%         j = j+1;
%         y_ref_merged(j) = u1(i); % u1
%         j = j+1;
%         y_ref_merged(j) = u1(i); % dt_u1
%         j = j+1;
%         y_ref_merged(j) = u1(i); % u2
%         j = j+1;
%         y_ref_merged(j) = u1(i); % u3
%         j = j+1;
    end

== matlab function Offline_MiL_Sim_Public/Vehicle Model/Thermisches Modell EM - LPTN/Subsystem1/MATLAB Function ==
  data: speed input; P_Iron_Mot output; torque input
function P_Iron_Mot = fcn(speed, torque)
% meanx_iron, meanx_current, meanx_frict, stdx_iron, stdx_current,...
%     stdx_frict, meany_iron, meany_current, meany_frict, stdy_iron, stdy_current, stdy_frict]
% Moteral:
% The idea is that the x variable is replaced by (x-mean(x))/std(x) and the y variable is
% replace similarly. This is done before any polynomial terms are computed. The transformation
% won't change the fit theoretically, but it will make the results better
% conditioned on a computer with finite precision.

% x: v, y:M_EM_acc, z:M_EM_brk

meanx_mot = 6252;
stdx_mot = 3696;
meany_mot = 67.04;
stdy_mot = 49.49;
x_rpm = speed;
x_scaled =  (x_rpm-meanx_mot)/stdx_mot ;
y_scaled = (torque-meany_mot)/stdy_mot;

p00_i =       970.5; 
p10_i =        1203;  
p01_i =       867.6; 
p20_i =       559.9; 
p11_i =       958.9;
p02_i =       200.2;
p21_i =         362;
p12_i =       170.7;
p03_i =      -15.11;
P_Iron_Mot = p00_i + p10_i*x_scaled + p01_i*y_scaled + p20_i*x_scaled^2 + p11_i*x_scaled*y_scaled + p02_i*y_scaled^2 + p21_i*(x_scaled^2)*y_scaled + p12_i*x_scaled*y_scaled^2 + p03_i*y_scaled^3;

== matlab function Offline_MiL_Sim_Public/Distance Check/Distance Change Security Check/MATLAB Function ==
  data: s input; bool_stop output; s_old input; start_distance_check input; break_criteria input
function bool_stop = distance_check(s,s_old, start_distance_check, break_criteria)
% start_distance_check in meters
% break_criteria in meters

if s  >= start_distance_check
    if (s-s_old) <= break_criteria
        bool_stop = 1;
    else
        bool_stop = 0;
    end
else
    bool_stop = 0;
end

== matlab function Offline_MiL_Sim_Public/Vehicle Model/Thermisches Modell EM - LPTN/Subsystem2/MATLAB Function ==
  data: speed input; P_Frict_Mot output; torque input
function P_Frict_Mot = fcn(speed, torque)
% meanx_iron, meanx_current, meanx_frict, stdx_iron, stdx_current,...
%     stdx_frict, meany_iron, meany_current, meany_frict, stdy_iron, stdy_current, stdy_frict]
% Moteral:
% The idea is that the x variable is replaced by (x-mean(x))/std(x) and the y variable is
% replace similarly. This is done before any polynomial terms are computed. The transformation
% won't change the fit theoretically, but it will make the results better
% conditioned on a computer with finite precision.

% x: v, y:M_EM_acc, z:M_EM_brk

meanx_mot = 6252;
stdx_mot = 3696;
meany_mot = 67.04;
stdy_mot = 49.49;

abs_torque = abs(torque);

x_rpm = speed;
x_scaled =  (x_rpm-meanx_mot)/stdx_mot ;
y_scaled = (abs_torque-meany_mot)/stdy_mot;

p00_f =       437.7;
p10_f =         348;
p01_f =       -8.25;
P_Frict_Mot = p00_f + p10_f*x_scaled + p01_f*y_scaled;

if torque <0
    P_Frict_Mot = -1 * P_Frict_Mot;
end

== matlab function Offline_MiL_Sim_Public/Reference Trajectory/distance preview ==
  data: v_ist input; s_ist input; a_ist input; s_prev output; Ts input; p_hor input; s_matrix input; v_prev_old input; delta_v_matrix input; t_in input; a_prev output
function [s_prev,a_prev] = preview_dist(v_ist,s_ist,a_ist,Ts,p_hor,s_matrix,v_prev_old,delta_v_matrix,t_in)
%#codegen
%Initialisierung
s_out = s_matrix;
a = s_matrix;
deltav = delta_v_matrix;


deltav = diff(v_prev_old)';
% s_ist = s_ist+1;

if t_in >1
    a(1) = a_ist;
    a(2:end-1) = deltav(2:end)/Ts;
    a(end) = deltav(end)/Ts;
    %         a(1:end-1) = deltav(1:end)/Ts;
    %         a(end) = deltav(end)/Ts;
end
if t_in <1
    %     a(1:end-1) = deltav(1:end)/Ts;
    %     a(end) = deltav(end)/Ts;
    a(:) = a_ist;
end

for i=1:p_hor
    s_out(i) = s_ist+Ts*v_ist+1/2*a(i)*Ts^2;
    v = v_ist + a(i)*Ts;
    v_ist = v;
    s_ist = s_out(i);
end
% ds = s_out(end)-s_out(end-1);
% s_out(1:end-1) = s_out(1:end);
% s_out(end) = s_out(end-1)+ds;
ds = s_out(end)-s_out(end-1);
s_out(1:end-4) = s_out(5:end);
s_out(end-3:end) = s_out(end-4)+[ds,2*ds,3*ds,4*ds];

a_prev = a;
a_prev(1:end-1) = a(2:end); % shift a_prev, s.t. a(1) = a_k+1
a_prev(end) = a(end);
s_prev = s_out;

== matlab function Offline_MiL_Sim_Public/Vehicle Model/Thermisches Modell EM - LPTN/Subsystem3/MATLAB Function ==
  data: speed input; P_Current_Mot output; torque input
function P_Current_Mot = fcn(speed, torque)
% meanx_iron, meanx_current, meanx_frict, stdx_iron, stdx_current,...
%     stdx_frict, meany_iron, meany_current, meany_frict, stdy_iron, stdy_current, stdy_frict]
% Moteral:
% The idea is that the x variable is replaced by (x-mean(x))/std(x) and the y variable is
% replace similarly. This is done before any polynomial terms are computed. The transformation
% won't change the fit theoretically, but it will make the results better
% conditioned on a computer with finite precision.

% x: v, y:M_EM_acc, z:M_EM_brk

meanx_mot = 6252;
stdx_mot = 3696;
meany_mot = 67.04;
stdy_mot = 49.49;
x_rpm = speed;
x_scaled =  (x_rpm-meanx_mot)/stdx_mot ;
y_scaled = (torque-meany_mot)/stdy_mot;

p00_c =        1172;  
p10_c =       785.1;  
p01_c =        1868;  
p20_c =       555.3; 
p11_c =       937.4;  
p02_c =         673; 
p21_c =       513.8;  
p12_c =       242.1;
p03_c =        -129;
P_Current_Mot = p00_c + p10_c*x_scaled + p01_c*y_scaled + p20_c*x_scaled^2 + p11_c*x_scaled*y_scaled + p02_c*y_scaled^2 + p21_c*(x_scaled^2)*y_scaled + p12_c*x_scaled*y_scaled^2 + p03_c*y_scaled^3;

== matlab function Offline_MiL_Sim_Public/MPC/MATLAB Function ==
  data: x input; y_ref_merged output; u1 input; P input
function y_ref_merged = get_ref_traj(x,u1,P)
%#codegen
%     y_ref_merged = zeros(150,1);
%     y_ref_merged = zeros(P*(n_controls-2+n_states),1);
    j = 1;
    % Depended on: y _ [v, M_EM_acc, M_EM_brk, M-fric_brk];
    
    y_ref_merged = zeros(160,1);
    for i=1:P
        y_ref_merged(j) = x(i); % v
        j = j+1;
        y_ref_merged(j) = u1(i); % u1
        j = j+1;
        y_ref_merged(j) = u1(i); % u2
        j = j+1;
        y_ref_merged(j) = u1(i); % u3
        j = j+1;
%         y_ref_merged(j) = x(i); % v
%         j = j+1;
%         y_ref_merged(j) = u1(i); % u1
%         j = j+1;
%         y_ref_merged(j) = u1(i); % dt_u1
%         j = j+1;
%         y_ref_merged(j) = u1(i); % u2
%         j = j+1;
%         y_ref_merged(j) = u1(i); % u3
%         j = j+1;
    end

== matlab function Offline_MiL_Sim_Public/MPC/SolverStop/MATLAB Function ==
  data: solver_status input; bool_stop output
function bool_stop = solver_status_check(solver_status)
% start_distance_check in meters
% break_criteria in meters

if solver_status  == 4
    bool_stop = 1;
else
    bool_stop = 0;
end

== matlab function Offline_MiL_Sim_Public/MPC/Pred_Traj_and_costs_calc/Subsystem/MATLAB Function ==
  data: v input; v_ref input; u input; cost output; dt_u input; Q input; R input; U input; cost_Q output; cost_R output; cost_U output; cost_traj output; P input
function [cost, cost_Q, cost_R, cost_U, cost_traj] = calc_costs(v, v_ref, u, dt_u, Q, R, U, P)
%#codegen
% cost = 0;
cost_Q = 0;
cost_U = 0;
cost_R = 0;
% cost_traj = zeros(30);
for i=1:P
    cost_Q = cost_Q + (v(i)-v_ref(i))^2*Q;
    cost_U = cost_U + u(i)^2*R ;
    cost_R = cost_R + dt_u(i)^2*U; 
end
cost = cost_Q + cost_R + cost_U;
cost_traj = (v-v_ref).*(v-v_ref)*Q + u.*u*R + dt_u.*dt_u*U;
